simulink model "filter"  (R2015a)
settings: Solver=ode45  StartTime=0.0  StopTime=10.0  RelTol=1e-3
libraries: dsparch4 x1, commnoisgen2 x1
settings Model: Creator=nikit  LastModifiedBy=nikit

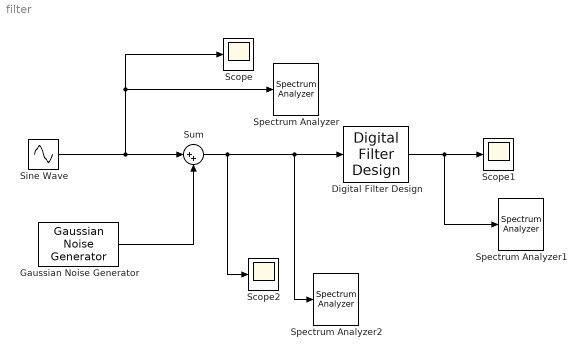
== system filter ==
  Digital Filter Design : dsparch4/Digital Filter Design  mwdsp_browser_bugfix_var=off
  Gaussian Noise Generator : commnoisgen2/Gaussian Noise Generator  m=0  d=1  s=41  Ts=1/1000  frameBased=off  sampPerFrame=1  orient=off  outDataType=single
  Scope : Scope
  Scope1 : Scope
  Scope2 : Scope
      settings: SaveName=ScopeData2
  Sine Wave : Sin  Amplitude=7  Frequency=50  Phase=7  SampleTime=1/1000
  Spectrum Analyzer : SpectrumAnalyzer
  Spectrum Analyzer1 : SpectrumAnalyzer
  Spectrum Analyzer2 : SpectrumAnalyzer
  Sum : Sum  Inputs=|++
  wires:
  Sine Wave/1 -> Spectrum Analyzer/1, Scope/1, Sum/1
  Sum/1 -> Scope2/1, Spectrum Analyzer2/1, Digital Filter Design/1
  Gaussian Noise Generator/1 -> Sum/2
  Digital Filter Design/1 -> Spectrum Analyzer1/1, Scope1/1
